simulink model "RollAngleController"  (Simulink 8.5)
settings: Solver=ode45  StartTime=0  StopTime=50.0  FixedStep=1  RelTol=1e-3
libraries: simulink x4
settings Model: Creator=Suriya  LastModifiedBy=spachaimuthu
settings DebuggingCC: SolverPrmCheckMsg=warning  FcnCallInpInsideContextMsg=EnableAllAsWarning
settings GRTTargetCC: CombineOutputUpdateFcns=on  GRTInterface=off

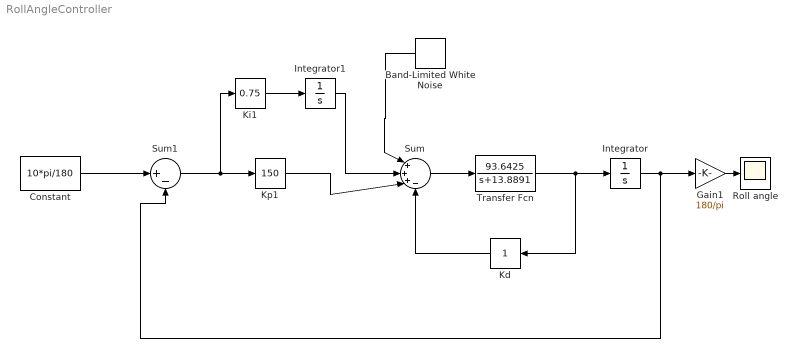
== system RollAngleController ==
  Band-Limited White Noise : simulink/Sources/Band-Limited White Noise  Cov=[0.1]  Ts=0.1  seed=[23341]
  Constant : Constant  Value=10*pi/180
  Gain1 : Gain  Gain=180/pi
  Integrator : Integrator
  Integrator1 : Integrator
  Kd : simulink/Math Operations/Slider Gain  low=0  gain=1  high=10
  Ki1 : simulink/Math Operations/Slider Gain  low=0  gain=0.75  high=200
  Kp1 : simulink/Math Operations/Slider Gain  low=0  gain=150  high=500
  Roll angle : Scope
  Sum : Sum  Inputs=|+++-
  Sum1 : Sum  Inputs=|+-
  Transfer Fcn : TransferFcn  Numerator=[93.6425]  Denominator=[1 13.8891]
  wires:
  Sum/1 -> Transfer Fcn/1
  Ki1/1 -> Integrator1/1
  Transfer Fcn/1 -> Integrator/1, Kd/1
  Band-Limited White Noise/1 -> Sum/1
  Integrator1/1 -> Sum/2
  Kp1/1 -> Sum/3
  Kd/1 -> Sum/4
  Sum1/1 -> Kp1/1, Ki1/1
  Integrator/1 -> Gain1/1, Sum1/2
  Constant/1 -> Sum1/1
  Gain1/1 -> Roll angle/1
